simulink library "app"  (R2021b)
settings: Solver=VariableStepAuto  StartTime=0.0  StopTime=10.0  RelTol=1e-3
undefined symbols (not defined in the file): C_TASK_10MS_S, C_TASK_5MS_S, slcm
libraries: acc x1, apm x1, bcm x1, ddm x1, dhp x1, did x1, dkc x1, dsc x1, nmm x1, pmm x1, psa x1, scp x1
settings Model: Creator=jc19  LastModifiedBy=zack
settings SolverCC: AlgebraicLoopSolver=TrustRegion
settings DataIOCC: SaveFormat=Array  SignalLoggingSaveFormat=ModelDataLogs  ReturnWorkspaceOutputs=off
settings OptimizationCC: BlockReduction=off  BooleanDataType=off
settings DebuggingCC: SaveWithParameterizedLinksMsg=none  UnderspecifiedInitializationDetection=Classic  MergeDetectMultiDrivingBlocksExec=none  SignalResolutionControl=TryResolveAllWithWarning  SFMachineParentedDataDiag=warning
settings HardwareCC: TargetUnknown=on
settings ModelReferenceCC: PropagateSignalLabelsOutOfModel=off
settings SFSimCC: SimUseLocalCustomCode=off
settings RTWCC: RTWUseLocalCustomCode=off
settings ConfigComp: CovMetricSettings=dw  CovSaveCumulativeToWorkspaceVar=on  CovSaveSingleToWorkspaceVar=on

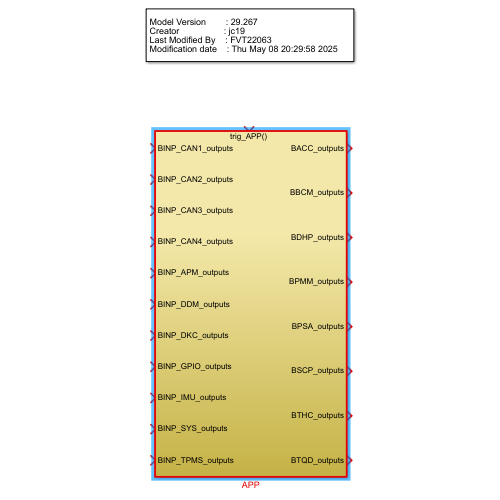
[thumbnail: Simulink's stored preview of the top-level diagram]
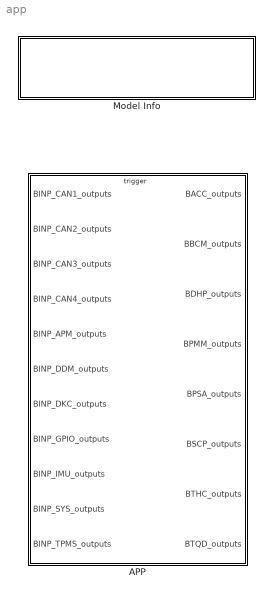
== system app ==
  APP : Subsystem
  Model Info : Subsystem  LoadFcn=slcm LoadBlock;  InitFcn=slcm('UpdateAllCMBlocksInThisModelInit')  mask(CMBlock){InitialSaveTempField=, InitialBlockCM=None, BlockCM=None, Frame=on, SaveTempField=, DisplayStringWithTags=|, MaskDisplayString=Model Version        : 29.271\nCreator                  : jc19\nLast Modified By    : zack\nModification date    : Mon May 26 17:49:11 2025, HorizontalTextAlignment=Left, LeftAlignmentValue=0.02, SourceBlockDiagram=app, TagMaxNumber=20, CMTag1=, CMTag2=, CMTag3=, CMTag4=, CMTag5=, CMTag6=, CMTag7=, CMTag8=, CMTag9=, CMTag10=, CMTag11=, CMTag12=, CMTag13=, CMTag14=, CMTag15=, CMTag16=, CMTag17=, CMTag18=, CMTag19=, CMTag20=}
      mask DisplayStringWithTags=|
      | Model Version        : %<ModelVersion>
      | Creator                  : %<Creator>
      | Last Modified By    : %<LastModifiedBy>
      | Modification date    : %<LastModificationDate>
      mask help: This block allows revision control information to be displayed within the model.
      settings: CopyFcn=slcm CopyBlock;  DeleteFcn=slcm Cancel;  PostSaveFcn=slcm('UpdateAllCMBlocksInThisModel')  NameChangeFcn=slcm Rename;  OpenFcn=slcm
      mask Display: text(str2num(LeftAlignmentValue), 0.5, MaskDisplayString, 'HorizontalAlignment', HorizontalTextAlignment)

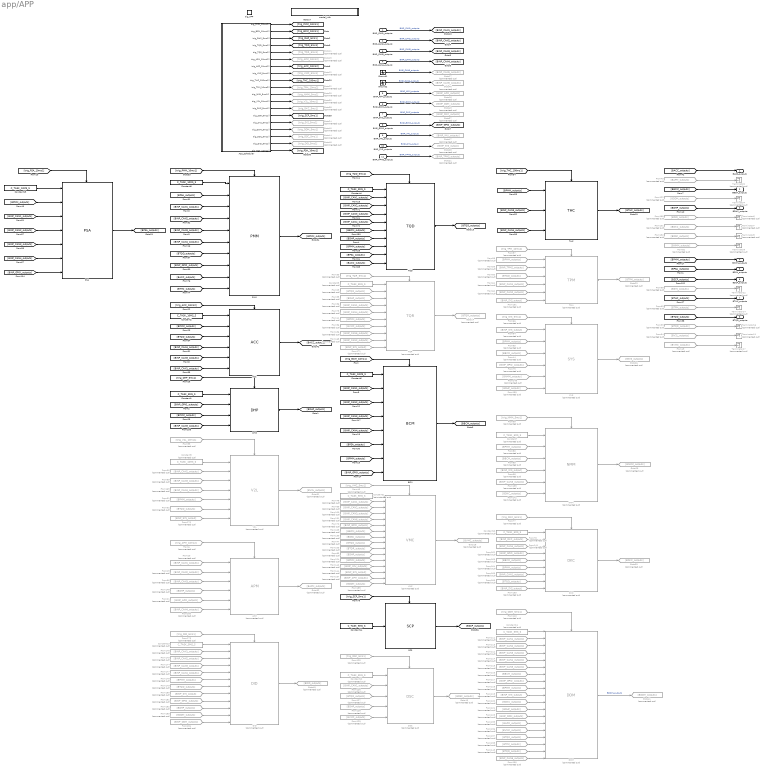
== system app/APP ==
  BINP_CAN1_outputs : Inport  OutDataTypeStr=Bus: BINP_CAN1_outputs
  BINP_CAN2_outputs : Inport  Port=2  OutDataTypeStr=Bus: BINP_CAN2_outputs
  BINP_CAN3_outputs : Inport  Port=3  OutDataTypeStr=Bus: BINP_CAN3_outputs
  BINP_CAN4_outputs : Inport  Port=4  OutDataTypeStr=Bus: BINP_CAN4_outputs
  BINP_APM_outputs : Inport  Port=5  OutDataTypeStr=Bus: BINP_APM_outputs
  BINP_DDM_outputs : Inport  Port=6  OutDataTypeStr=Bus: BINP_DDM_outputs
  BINP_DKC_outputs : Inport  Port=7  OutDataTypeStr=Bus: BINP_DKC_outputs
  BINP_GPIO_outputs : Inport  Port=8  OutDataTypeStr=Bus: BINP_GPIO_outputs
  BINP_IMU_outputs : Inport  Port=9  OutDataTypeStr=Bus: BINP_IMU_outputs
  BINP_SYS_outputs : Inport  Port=10  OutDataTypeStr=Bus: BINP_SYS_outputs
  BINP_TPMS_outputs : Inport  Port=11  OutDataTypeStr=Bus: BINP_TPMS_outputs
  trig_APP : TriggerPort  TriggerType=function-call  VariantControl=(inherit)
  ACC : acc/ACC  SystemSampleTime=-1  VariantActivationTime=update diagram  Latency=0  AutoFrameSizeCalculation=off
  APM : apm/APM  Commented=on  SystemSampleTime=-1  VariantActivationTime=update diagram  Latency=0  AutoFrameSizeCalculation=off
  App_Scheduler : Stateflow chart  TreatAsAtomicUnit=on
  BCM : bcm/BCM  SystemSampleTime=-1  VariantActivationTime=update diagram  Latency=0  AutoFrameSizeCalculation=off
  Constant1 : Constant  Value=C_TASK_5MS_S  OutDataTypeStr=single
  Constant{3,5,7,10..13} (7 alike) : Constant  Commented=on  Value=C_TASK_5MS_S  OutDataTypeStr=single
  Constant14 : Constant  Value=C_TASK_5MS_S  OutDataTypeStr=single
  Constant{2,6,8,15} (4 alike) : Constant  Value=C_TASK_10MS_S  OutDataTypeStr=single
  Constant4 : Constant  Value=C_TASK_5MS_S  OutDataTypeStr=single
  Constant9 : Constant  Commented=on  Value=C_TASK_10MS_S  OutDataTypeStr=single
  DDM : ddm/DDM  Commented=on  SystemSampleTime=-1  VariantActivationTime=update diagram  Latency=0  AutoFrameSizeCalculation=off
  DHP : dhp/DHP  SystemSampleTime=-1  VariantActivationTime=update diagram  Latency=0  AutoFrameSizeCalculation=off
  DID : did/DID  Commented=on  SystemSampleTime=-1  VariantActivationTime=update diagram  Latency=0  AutoFrameSizeCalculation=off
  DKC : dkc/DKC  Commented=on  SystemSampleTime=-1  VariantActivationTime=update diagram  Latency=0  AutoFrameSizeCalculation=off
  DSC : dsc/DSC  Commented=on  SystemSampleTime=-1  VariantActivationTime=update diagram  Latency=0  AutoFrameSizeCalculation=off
  From{86,89,100,112,139,174} (6 alike) : From  Commented=on  GotoTag=BINP_CAN3_outputs
  From101 : From  Commented=on  GotoTag=BDKC_outputs
  From103 : From  Commented=on  GotoTag=BTQR_outputs
  From{44,85,109,116,163} (5 alike) : From  Commented=on  GotoTag=BBCM_outputs
  From110 : From  Commented=on  GotoTag=trig_DDM_5ms1
  From{20,36,48,61,111,126,165,176} (8 alike) : From  Commented=on  GotoTag=BINP_CAN1_outputs
  From{19,62,69,90,113,168,175} (7 alike) : From  Commented=on  GotoTag=BINP_CAN2_outputs
  From{73,114,141,160,169,177} (6 alike) : From  Commented=on  GotoTag=BINP_CAN4_outputs
  From115 : From  Commented=on  GotoTag=BINP_CAN5_outputs
  From{70,75,117,162,181} (5 alike) : From  Commented=on  GotoTag=BINP_GPIO_outputs
  From{41,58,65,80,91,118,124,164,178} (9 alike) : From  Commented=on  GotoTag=BPMM_outputs
  From{84,98,119,144,170..171,180,191,193} (9 alike) : From  Commented=on  GotoTag=BINP_SYS_output
  From120 : From  Commented=on  GotoTag=BDKC_outputs
  From{35,83,121,128,148,159,182} (7 alike) : From  Commented=on  GotoTag=BDHP_outputs
  From122 : From  Commented=on  GotoTag=BDDM_outputs
  From123 : From  Commented=on  GotoTag=BINP_DDM_outputs
  From125 : From  Commented=on  GotoTag=trig_DSC_5ms1
  From{29,47,60,92,127,143,166,179} (8 alike) : From  Commented=on  GotoTag=BTQD_outputs
  From{49,96,129,136} (4 alike) : From  Commented=on  GotoTag=BVMC_outputs
  From130 : From  Commented=on  GotoTag=BDSC_outputs
  From131 : From  Commented=on  GotoTag=BINP_CAN6_outputs
  From132 : From  Commented=on  GotoTag=BDSC_outputs
  From135 : From  Commented=on  GotoTag=BAPM_outputs
  From137 : From  Commented=on  GotoTag=BTQR_outputs
  From138 : From  Commented=on  GotoTag=BTPM_outputs
  From142 : From  Commented=on  GotoTag=BINP_IMU_outputs
  From145 : From  Commented=on  GotoTag=BNMM_outputs
  From156 : From  Commented=on  GotoTag=BINP_CAN6_outputs
  From167 : From  Commented=on  GotoTag=BINP_APM_outputs
  From172 : From  Commented=on  GotoTag=BDKC_outputs
  From173 : From  Commented=on  GotoTag=trig_DID_5ms1
  From183 : From  Commented=on  GotoTag=BDDM_outputs
  From184 : From  Commented=on  GotoTag=BINP_DDM_outputs
  From185 : From  Commented=on  GotoTag=BDID_outputs
  From189 : From  Commented=on  GotoTag=BDDM_outputs
  From190 : From  Commented=on  GotoTag=BINP_CAN6_outputs
  From21 : From  Commented=on  GotoTag=BINP_APM_outputs
  From33 : From  Commented=on  GotoTag=trig_TQR_5ms1
  From39 : From  Commented=on  GotoTag=BTQR_outputs
  From43 : From  Commented=on  GotoTag=BAPM_outputs
  From46 : From  Commented=on  GotoTag=trig_VMC_5ms1
  From57 : From  Commented=on  GotoTag=trig_TPM_10ms2
  From59 : From  Commented=on  GotoTag=BINP_TPMS_outputs
  From6 : From  Commented=on  GotoTag=trig_APM_10ms2
  From63 : From  Commented=on  GotoTag=BTPM_outputs
  From66 : From  Commented=on  GotoTag=trig_SYS_5ms1
  From68 : From  Commented=on  GotoTag=BSYS_outputs
  From77 : From  Commented=on  GotoTag=trig_DKC_5ms1
  From78 : From  Commented=on  GotoTag=BINP_DKC_outputs
  From82 : From  Commented=on  GotoTag=BNMM_outputs
  From93 : From  Commented=on  GotoTag=trig_V2L_10ms1
  From94 : From  Commented=on  GotoTag=BV2L_outputs
  From99 : From  Commented=on  GotoTag=trig_NMM_5ms1
  Goto11 : Goto  Commented=on  GotoTag=trig_TQR_5ms1
  Goto12 : Goto  Commented=on  GotoTag=trig_VMC_5ms1
  Goto14 : Goto  Commented=on  GotoTag=BTQR_outputs
  Goto15 : Goto  Commented=on  GotoTag=trig_APM_10ms2
  Goto16 : Goto  Commented=on  GotoTag=BINP_APM_outputs
  Goto17 : Goto  Commented=on  GotoTag=BINP_CAN5_outputs
  Goto18 : Goto  Commented=on  GotoTag=BVMC_outputs
  Goto21 : Goto  Commented=on  GotoTag=BINP_TPMS_outputs
  Goto22 : Goto  Commented=on  GotoTag=trig_TPM_10ms2
  Goto23 : Goto  Commented=on  GotoTag=BTPM_outputs
  Goto24 : Goto  Commented=on  GotoTag=trig_SYS_5ms1
  Goto25 : Goto  Commented=on  GotoTag=trig_NMM_5ms1
  Goto26 : Goto  Commented=on  GotoTag=BSYS_outputs
  Goto28 : Goto  Commented=on  GotoTag=BINP_SYS_output
  Goto29 : Goto  Commented=on  GotoTag=BNMM_outputs
  Goto30 : Goto  Commented=on  GotoTag=trig_V2L_10ms1
  Goto31 : Goto  Commented=on  GotoTag=BV2L_outputs
  Goto32 : Goto  Commented=on  GotoTag=BAPM_outputs
  Goto37 : Goto  Commented=on  GotoTag=BINP_DKC_outputs
  Goto38 : Goto  Commented=on  GotoTag=trig_DKC_5ms1
  Goto39 : Goto  Commented=on  GotoTag=BDKC_outputs
  Goto40 : Goto  Commented=on  GotoTag=trig_DDM_5ms1
  Goto41 : Goto  Commented=on  GotoTag=BDDM_outputs
  Goto43 : Goto  Commented=on  GotoTag=BINP_DDM_outputs
  Goto44 : Goto  Commented=on  GotoTag=trig_DSC_5ms1
  Goto45 : Goto  Commented=on  GotoTag=BDSC_outputs
  Goto46 : Goto  Commented=on  GotoTag=BINP_CAN6_outputs
  Goto47 : Goto  Commented=on  GotoTag=BINP_IMU_outputs
  Goto48 : Goto  Commented=on  GotoTag=trig_DID_5ms1
  Goto49 : Goto  Commented=on  GotoTag=BDID_outputs
  Ground1 : Ground
  Ground2 : Ground
  NMM : nmm/NMM  Commented=on  SystemSampleTime=-1  VariantActivationTime=update diagram  Latency=0  AutoFrameSizeCalculation=off
  PMM : pmm/PMM  SystemSampleTime=-1  VariantActivationTime=update diagram  Latency=0  AutoFrameSizeCalculation=off
  PSA : psa/PSA  SystemSampleTime=-1  VariantActivationTime=update diagram  Latency=0  AutoFrameSizeCalculation=off
  SCP : scp/SCP  SystemSampleTime=-1  VariantActivationTime=update diagram  Latency=0  AutoFrameSizeCalculation=off
  SYS : sys/SYS  Commented=on  SystemSampleTime=-1  VariantActivationTime=update diagram  Latency=0  AutoFrameSizeCalculation=off
  THC : thc/THC  SystemSampleTime=-1  VariantActivationTime=update diagram  Latency=0  AutoFrameSizeCalculation=off
  TPM : tpm/TPM  Commented=on  SystemSampleTime=-1  VariantActivationTime=update diagram  Latency=0  AutoFrameSizeCalculation=off
  TQD : tqd/TQD  SystemSampleTime=-1  VariantActivationTime=update diagram  Latency=0  AutoFrameSizeCalculation=off
  TQR : tqr/TQR  Commented=on  SystemSampleTime=-1  VariantActivationTime=update diagram  Latency=0  AutoFrameSizeCalculation=off
  Terminator{2,4,6..9,11..12,14,16..17} (11 alike) : Terminator  Commented=on
  V2L : v2l/V2L  Commented=on  SystemSampleTime=-1  VariantActivationTime=update diagram  Latency=0  AutoFrameSizeCalculation=off
  VMC : vmc/VMC  Commented=on  SystemSampleTime=-1  VariantActivationTime=update diagram  Latency=0  AutoFrameSizeCalculation=off
  model_info : Subsystem  LoadFcn=slcm LoadBlock;  InitFcn=slcm('UpdateAllCMBlocksInThisModelInit')  mask(CMBlock){InitialSaveTempField=, InitialBlockCM=None, BlockCM=None, Frame=on, SaveTempField=, DisplayStringWithTags=$Id: app.mdl 2023 2013-03-20 03:40:02Z wxia $, MaskDisplayString=$Id: app.mdl 2023 2013-03-20 03:40:02Z wxia $, HorizontalTextAlignment=Center, LeftAlignmentValue=0.5, SourceBlockDiagram=app, TagMaxNumber=20, CMTag1=, CMTag2=, CMTag3=, CMTag4=, CMTag5=, CMTag6=, CMTag7=, CMTag8=, CMTag9=, CMTag10=, CMTag11=, CMTag12=, CMTag13=, CMTag14=, CMTag15=, CMTag16=, CMTag17=, CMTag18=, CMTag19=, CMTag20=}
      mask help: This block allows revision control information to be displayed within the model.
      settings: CopyFcn=slcm CopyBlock;  DeleteFcn=slcm Cancel;  PostSaveFcn=slcm('UpdateAllCMBlocksInThisModel')  NameChangeFcn=slcm Rename;  OpenFcn=slcm
      mask Display: text(str2num(LeftAlignmentValue), 0.5, MaskDisplayString, 'HorizontalAlignment', HorizontalTextAlignment)
  BACC_outputs : Outport  OutDataTypeStr=Bus: BACC_outputs  VectorParamsAs1DForOutWhenUnconnected=off
  BBCM_outputs : Outport  Port=2  OutDataTypeStr=Bus: BBCM_outputs  VectorParamsAs1DForOutWhenUnconnected=off
  BDHP_outputs : Outport  Port=3  OutDataTypeStr=Bus: BDHP_outputs  VectorParamsAs1DForOutWhenUnconnected=off
  BPMM_outputs : Outport  Port=4  OutDataTypeStr=Bus: BPMM_outputs  VectorParamsAs1DForOutWhenUnconnected=off
  BPSA_outputs : Outport  Port=5  OutDataTypeStr=Bus: BPSA_outputs  VectorParamsAs1DForOutWhenUnconnected=off
  BSCP_outputs : Outport  Port=6  OutDataTypeStr=Bus: BSCP_outputs  VectorParamsAs1DForOutWhenUnconnected=off
  BTHC_outputs : Outport  Port=7  OutDataTypeStr=Bus: BTHC_outputs  VectorParamsAs1DForOutWhenUnconnected=off
  BTQD_outputs : Outport  Port=8  OutDataTypeStr=Bus: BTQD_outputs  VectorParamsAs1DForOutWhenUnconnected=off
  wires:
  NMM/1 -> Goto29/1
  From99/1 -> NMM/Trigger
  Constant7/1 -> NMM/1
  DHP/1 -> [BDHP_outputs]
  Constant1/1 -> DHP/1
  [BINP_GPIO_outputs] -> DHP/2
  BINP_CAN1_outputs/1 -> [BINP_CAN1_outputs]  "BINP_CAN1_outputs"
  PMM/1 -> [BPMM_outputs]
  ACC/1 -> [BACC_outputs]
  [trig_PMM_10ms1] -> PMM/Trigger
  TQD/1 -> [BTQD_outputs]
  TQR/1 -> Goto14/1
  From29/1 -> TQR/2
  Constant2/1 -> ACC/1
  [trig_BCM_10ms1] -> BCM/Trigger
  BCM/1 -> [BBCM_outputs]
  BINP_CAN2_outputs/1 -> [BINP_CAN2_outputs]  "BINP_CAN2_outputs"
  BINP_CAN3_outputs/1 -> [BINP_CAN3_outputs]  "BINP_CAN3_outputs"
  BINP_CAN4_outputs/1 -> [BINP_CAN4_outputs]  "BINP_CAN4_outputs"
  BINP_GPIO_outputs/1 -> [BINP_GPIO_outputs]  "BINP_GPIO_outputs"
  [trig_TQD_5ms1] -> TQD/Trigger
  [BPMM_outputs] -> DHP/3
  [trig_DHP_5ms1] -> DHP/Trigger
  Ground1/1 -> Goto17/1  "BINP_CAN5_outputs"
  From33/1 -> TQR/Trigger
  Constant3/1 -> TQR/1
  From35/1 -> TQR/3
  From36/1 -> TQR/4
  [trig_ACC_10ms2] -> ACC/Trigger
  [BPMM_outputs] -> ACC/2
  From46/1 -> VMC/Trigger
  Constant5/1 -> VMC/1
  VMC/1 -> Goto18/1
  THC/1 -> [BTHC_outputs]
  [BPMM_outputs] -> THC/1
  [trig_THC_100ms1] -> THC/Trigger
  BINP_TPMS_outputs/1 -> Goto21/1  "BINP_TPMS_outputs"
  From57/1 -> TPM/Trigger
  From58/1 -> TPM/1
  From59/1 -> TPM/2
  From60/1 -> TPM/3
  From61/1 -> TPM/4
  From62/1 -> TPM/5
  TPM/1 -> Goto23/1
  SYS/1 -> Goto26/1
  From73/1 -> TQR/5
  From41/1 -> TQR/6
  BINP_SYS_outputs/1 -> Goto28/1  "BINP_SYS_output"
  Constant9/1 -> V2L/1
  From89/1 -> V2L/3
  From90/1 -> V2L/2
  From93/1 -> V2L/Trigger
  V2L/1 -> Goto31/1
  APM/1 -> Goto32/1
  From6/1 -> APM/Trigger
  From20/1 -> APM/1
  From19/1 -> APM/2
  BINP_APM_outputs/1 -> Goto16/1  "BINP_APM_outputs"
  From66/1 -> SYS/Trigger
  From86/1 -> APM/3
  From96/1 -> TQR/7
  Constant8/1 -> PMM/1
  From80/1 -> NMM/2
  From85/1 -> NMM/3
  From98/1 -> NMM/4
  App_Scheduler/3(trig_DHP_5ms1()) -> [trig_DHP_5ms1]
  App_Scheduler/4(trig_TQD_5ms1()) -> [trig_TQD_5ms1]
  App_Scheduler/8(trig_VMC_5ms1()) -> Goto12/1
  App_Scheduler/15(trig_SYS_5ms1()) -> Goto24/1
  App_Scheduler/2(trig_BCM_10ms1()) -> [trig_BCM_10ms1]
  App_Scheduler/12(trig_V2L_10ms1()) -> Goto30/1
  App_Scheduler/5(trig_TQR_5ms1()) -> Goto11/1
  App_Scheduler/9(trig_THC_100ms1()) -> [trig_THC_100ms1]
  App_Scheduler/6(trig_APM_10ms2()) -> Goto15/1
  App_Scheduler/7(trig_ACC_10ms2()) -> [trig_ACC_10ms2]
  App_Scheduler/11(trig_NMM_5ms1()) -> Goto25/1
  App_Scheduler/10(trig_TPM_10ms2()) -> Goto22/1
  App_Scheduler/1(trig_PMM_10ms1()) -> [trig_PMM_10ms1]
  App_Scheduler/13(trig_DKC_5ms1()) -> Goto38/1
  App_Scheduler/14(trig_SCP_5ms1()) -> [trig_SCP_5ms1]
  BINP_DKC_outputs/1 -> Goto37/1  "BINP_DKC_outputs"
  From77/1 -> DKC/Trigger
  Constant10/1 -> DKC/1
  From78/1 -> DKC/2
  SCP/1 -> [BSCP_outputs]
  DKC/1 -> Goto39/1
  From68/1 -> Terminator12/1
  From39/1 -> Terminator16/1
  From43/1 -> Terminator2/1
  [BPMM_outputs] -> BPMM_outputs/1
  From94/1 -> Terminator11/1
  [BTQD_outputs] -> BTQD_outputs/1
  [BDHP_outputs] -> BDHP_outputs/1
  From63/1 -> Terminator14/1
  From101/1 -> Terminator7/1
  [BACC_outputs] -> BACC_outputs/1
  From82/1 -> Terminator9/1
  From49/1 -> Terminator17/1
  [BSCP_outputs] -> BSCP_outputs/1
  [BBCM_outputs] -> BBCM_outputs/1
  [BTHC_outputs] -> BTHC_outputs/1
  From84/1 -> SYS/1
  From65/1 -> SYS/2
  From44/1 -> SYS/3
  From75/1 -> SYS/4
  App_Scheduler/16(trig_DDM_5ms1()) -> Goto40/1
  From110/1 -> DDM/Trigger
  From122/1 -> Terminator4/1
  BINP_DDM_outputs/1 -> Goto43/1  "BINP_DDM_outputs"
  From48/1 -> VMC/2
  From69/1 -> VMC/3
  From100/1 -> VMC/4
  App_Scheduler/17(trig_DSC_5ms1()) -> Goto44/1
  From125/1 -> DSC/Trigger
  Constant12/1 -> DSC/1
  From126/1 -> DSC/2
  From127/1 -> DSC/3
  From128/1 -> DSC/4
  From129/1 -> DSC/5
  DSC/1 -> Goto45/1
  Ground2/1 -> Goto46/1  "BINP_CAN6_outputs"
  From132/1 -> Terminator8/1
  Constant6/1 -> BCM/1
  Constant11/1 -> DDM/1
  From111/1 -> DDM/2
  From113/1 -> DDM/3
  From112/1 -> DDM/4
  From114/1 -> DDM/5
  From115/1 -> DDM/6
  From116/1 -> DDM/7
  From117/1 -> DDM/8
  From118/1 -> DDM/9
  From119/1 -> DDM/10
  From120/1 -> DDM/11
  From121/1 -> DDM/12
  From123/1 -> DDM/13
  From135/1 -> DDM/14
  From136/1 -> DDM/15
  From137/1 -> DDM/16
  From138/1 -> DDM/17
  From139/1 -> NMM/5
  [BINP_CAN3_outputs] -> THC/2
  [BINP_CAN4_outputs] -> THC/3
  From141/1 -> DKC/3
  DDM/1 -> Goto41/1  "BDDM_outputs"
  BINP_IMU_outputs/1 -> Goto47/1  "BINP_IMU_outputs"
  From143/1 -> DDM/18
  From145/1 -> SYS/5
  Constant4/1 -> TQD/1
  From21/1 -> APM/5
  From148/1 -> APM/4
  From131/1 -> VMC/5
  From70/1 -> VMC/6
  From109/1 -> VMC/7
  From130/1 -> VMC/8
  From47/1 -> VMC/9
  From103/1 -> VMC/10
  From83/1 -> VMC/11
  From124/1 -> VMC/12
  From142/1 -> VMC/13
  From144/1 -> VMC/14
  From156/1 -> TQR/8
  [BINP_CAN3_outputs] -> DHP/4
  From160/1 -> APM/6
  From162/1 -> DKC/4
  From163/1 -> DKC/5
  From164/1 -> DKC/6
  From165/1 -> DKC/7
  From166/1 -> DKC/8
  From167/1 -> VMC/15
  From168/1 -> TQR/9
  From92/1 -> V2L/6
  From91/1 -> V2L/5
  From169/1 -> V2L/4
  From170/1 -> V2L/7
  From159/1 -> SYS/6
  From171/1 -> TQR/10
  From172/1 -> NMM/6
  App_Scheduler/18(trig_DID_5ms1()) -> Goto48/1
  From173/1 -> DID/Trigger
  Constant13/1 -> DID/1
  From176/1 -> DID/2
  From175/1 -> DID/3
  From174/1 -> DID/4
  From177/1 -> DID/5
  From178/1 -> DID/6
  From179/1 -> DID/7
  From180/1 -> DID/8
  From181/1 -> DID/9
  From182/1 -> DID/10
  DID/1 -> Goto49/1
  From183/1 -> DID/11
  From184/1 -> DID/12
  From185/1 -> Terminator6/1
  From190/1 -> DDM/19
  From189/1 -> VMC/16
  From191/1 -> TPM/6
  From193/1 -> DKC/9
  Constant14/1 -> SCP/1
  [trig_SCP_5ms1] -> SCP/Trigger
  [BINP_CAN1_outputs] -> PMM/3
  [BINP_CAN2_outputs] -> PMM/4
  [BINP_CAN3_outputs] -> PMM/5
  [BINP_CAN4_outputs] -> PMM/6
  App_Scheduler/19(trig_PSA_10ms1()) -> [trig_PSA_10ms1]
  [trig_PSA_10ms1] -> PSA/Trigger
  PSA/1 -> [BPSA_outputs]
  [BPSA_outputs] -> PMM/2
  Constant15/1 -> PSA/1
  [BPMM_outputs] -> PSA/2
  [BINP_CAN1_outputs] -> PSA/3
  [BINP_CAN2_outputs] -> PSA/4
  [BINP_CAN3_outputs] -> PSA/5
  [BINP_CAN4_outputs] -> PSA/6
  [BPSA_outputs] -> BPSA_outputs/1
  [BINP_GPIO_outputs] -> PSA/7
  [BINP_CAN2_outputs] -> BCM/3
  [BINP_CAN1_outputs] -> BCM/2
  [BINP_CAN3_outputs] -> BCM/4
  [BINP_CAN4_outputs] -> BCM/5
  [BPSA_outputs] -> BCM/6
  [BPMM_outputs] -> BCM/7
  [BINP_GPIO_outputs] -> BCM/8
  [BINP_CAN1_outputs] -> TQD/2
  [BINP_CAN2_outputs] -> TQD/3
  [BINP_CAN3_outputs] -> TQD/4
  [BINP_CAN4_outputs] -> TQD/5
  [BBCM_outputs] -> TQD/6
  [BDHP_outputs] -> TQD/7
  [BPMM_outputs] -> TQD/8
  [BPSA_outputs] -> TQD/9
  [BTQD_outputs] -> PMM/7
  [BINP_GPIO_outputs] -> PMM/8
  [BINP_CAN3_outputs] -> ACC/5
  [BINP_CAN4_outputs] -> ACC/4
  [BINP_CAN1_outputs] -> ACC/6
  [BTQD_outputs] -> ACC/3
  [BACC_outputs] -> PMM/9
  [BTHC_outputs] -> PMM/10
  [BACC_outputs] -> TQD/10

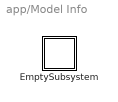
== system app/Model Info ==
  EmptySubsystem : Subsystem

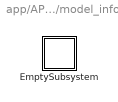
== system app/APP/model_info ==
  EmptySubsystem : Subsystem

== system app/Model Info/EmptySubsystem ==

== system app/APP/model_info/EmptySubsystem ==

== stateflow chart app/APP/App_Scheduler ==
  state Task_5_10_100ms
    (default) -> (junction 6) : {
        | counter = 0;
        | }
    Task_5_10_100ms -> (junction 6) : {
        | counter++;
        | }
    (junction 6) -> (junction 38) [order 1] : [counter%%2 == 0]  /* 10ms trigger #1*/
    (junction 6) -> (junction 44) [order 2]
    (junction 38) -> (junction 40) : {
        | trig_PSA_10ms1;
        | trig_PMM_10ms1;
        | trig_BCM_10ms1;
        | trig_V2L_10ms1;
        | }
    (junction 40) -> (junction 44)
    (junction 44) -> (junction 63)
    (junction 63) -> (junction 107) [order 1] : %[VPMM_PowerSta_enum == ENUM_POWERSTA_ON ||...
        | %VPMM_PowerSta_enum == ENUM_POWERSTA_READY]
    (junction 63) -> (junction 69) [order 2]
    (junction 107) -> (junction 108) : {
        | trig_DHP_5ms1;
        | trig_TQD_5ms1;
        | trig_TQR_5ms1;
        | trig_VMC_5ms1;
        | trig_NMM_5ms1;
        | trig_SCP_5ms1;
        | trig_DKC_5ms1;
        | trig_DSC_5ms1;
        | trig_DDM_5ms1;
        | trig_DID_5ms1;
        | }
    (junction 108) -> (junction 69)
    (junction 69) -> (junction 115)
    (junction 115) -> (junction 113) [order 1] : [counter%%2 == 1]  /* 10ms trigger #2*/
    (junction 115) -> (junction 124) [order 2]
    (junction 113) -> (junction 117) : {
        | trig_APM_10ms2;
        | trig_ACC_10ms2;
        | trig_TPM_10ms2;
        | }
    (junction 117) -> (junction 124)
    (junction 124) -> (junction 131)
    (junction 131) -> (junction 133) [order 1] : [counter%% 20 == 0]  /*100ms trigger #1*/
    (junction 131) -> (junction 137) [order 2]
    (junction 133) -> (junction 135) : {
        |  trig_THC_100ms1;
        |  counter = 0;
        |  }
    (junction 135) -> (junction 137)
    (junction 137) -> (junction 154) : {
        |  trig_SYS_5ms1;
        | }
  data: counter local double
  events: trig_PMM_10ms1 output FUNCTION_CALL_EVENT; trig_BCM_10ms1 output FUNCTION_CALL_EVENT; trig_DHP_5ms1 output FUNCTION_CALL_EVENT; trig_TQD_5ms1 output FUNCTION_CALL_EVENT; trig_TQR_5ms1 output FUNCTION_CALL_EVENT; trig_APM_10ms2 output FUNCTION_CALL_EVENT; trig_ACC_10ms2 output FUNCTION_CALL_EVENT; trig_VMC_5ms1 output FUNCTION_CALL_EVENT; trig_THC_100ms1 output FUNCTION_CALL_EVENT; trig_TPM_10ms2 output FUNCTION_CALL_EVENT; trig_NMM_5ms1 output FUNCTION_CALL_EVENT; trig_V2L_10ms1 output FUNCTION_CALL_EVENT; trig_DKC_5ms1 output FUNCTION_CALL_EVENT; trig_SCP_5ms1 output FUNCTION_CALL_EVENT; trig_SYS_5ms1 output FUNCTION_CALL_EVENT; trig_DDM_5ms1 output FUNCTION_CALL_EVENT; trig_DSC_5ms1 output FUNCTION_CALL_EVENT; trig_DID_5ms1 output FUNCTION_CALL_EVENT; trig_PSA_10ms1 output FUNCTION_CALL_EVENT
